simulink model "gm_fpga_block_pcie_slrt"  (R2020b)
settings: Solver=FixedStepDiscrete  StartTime=0.0  StopTime=5  FixedStep=5e-5  RelTol=1e-3
PostLoadFcn:
  | try
  | cell = struct2cell(dir(fullfile(speedgoatroot_hdlb, 'hdlsrc', 'quadrature', '*.vhd')));
  | addSourceFiles = strjoin(fullfile(cell(2,:),cell(1,:)), ';');
  | hdlset_param('quadrature_example_hdlc/DUT Quadrature', 'IPCoreAdditionalFiles', addSourceFiles);
  | end
undefined symbols (not defined in the file): FPGA, fpga_block, IO334
libraries: speedgoatlib_hdlCoder_IO3xx x19, eePwmGenerator x3, slrealtimeutilitieslib x1, pwm_cpulib x1, quadrature_cpulib x1
settings Model: ModifiedByFormat=Speedgoat GmbH  Creator=Speedgoat GmbH  LastModifiedBy=Speedgoat GmbH
settings SolverCC: ConcurrentTasks=on  PositivePriorityOrder=on
settings DataIOCC: ReturnWorkspaceOutputs=off
settings OptimizationCC: BlockReduction=off  ConditionallyExecuteInputs=off  DefaultParameterBehavior=Inlined  OptimizeBlockIOStorage=off
settings DebuggingCC: AlgebraicLoopMsg=error  InheritedTsInSrcMsg=none  SingleTaskRateTransMsg=error  TasksWithSamePriorityMsg=none  ParameterOverflowMsg=warning  ParameterPrecisionLossMsg=none  PregeneratedLibrarySubsystemCodeDiagnostic=none  ArithmeticOperatorsInVariantConditions=warning
settings HardwareCC: ProdBitPerLong=64  ProdLongLongMode=on  ProdHWDeviceType=Intel->x86-64 (Linux 64)  TargetBitPerPointer=64  TargetBitPerSizeT=64  TargetBitPerPtrDiffT=64  TargetLongLongMode=on  TargetIntDivRoundTo=Zero  TargetEndianess=LittleEndian  TargetWordSize=64  TargetHWDeviceType=Custom Processor->MATLAB Host Computer
settings SFSimCC: SimUseLocalCustomCode=off  CustomCodeUndefinedFunction=UseInterfaceOnly
settings RTWCC: Description=Simulink Real-Time  SystemTargetFile=slrealtime.tlc  TemplateMakefile=slrealtime_default_tmf  RTWUseLocalCustomCode=off  Toolchain=Simulink Real-Time Toolchain  BuildConfiguration=Faster Runs  CodeExecutionProfiling=on  TargetLang=C++

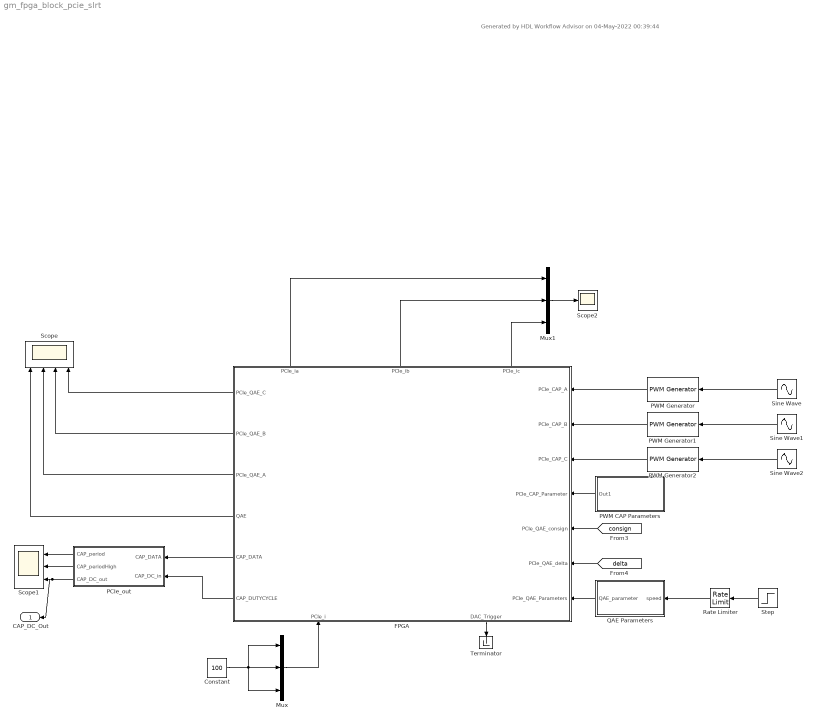
== system gm_fpga_block_pcie_slrt ==
  note: Generated by HDL Workflow Advisor on 04-May-2022 00:39:44
  Constant : Constant  Value=100  OutDataTypeStr=int16  SampleTime=5e-5
  FPGA : Subsystem  mask(Speedgoat IO334-325k Interface Block){module_id=1, slot=-1, ts=-1, FpgaFreq=100}
      mask prompts: module_id "FPGA Module Identifier:"; slot "PCI slot (-1: autosearch):"; ts "Sample time:"; FpgaFreq "FPGA Frequency [MHz]"
      mask help: Simulink Real-Time Interface Block for Speedgoat IO334-325k.
      mask init:
      | hdlslrt.backend.mfpgaparameters;
      settings: PortSchema="{\"entries\":[{\"content\":{\"sides\":[{\"content\":{\"connectorIds\":[\"In1\",\"In2\",\"In3\",\"In4\",\"In5\",\"In6\",\"In7\"]},\"type\":\"ConnectorPlacement.EquallySpacedRectSide\",\"uuid\":\"e6984190-0c70-4c87-a85a-93b5ecf8c70e\"},{\"content\":{\"connectorIds\":[\"Out1\",\"Out2\",\"Out3\",\"Out4\",\"Out5\",\"Out6\"],\"side\":\"RIGHT\"},\"type\":\"ConnectorPlacement.EquallySpacedRectSide\",\"uuid\":\"15751016-c591-4c93-a1ea-9b92ed7cff5f\"},{\"content\":{\"connectorIds\":[\"Out8\",\"Out9\",\"Out10\"],\"side\":\"TOP\"},\"type\":\"ConnectorPlacement.EquallySpacedRectSide\",\"uuid\":\"0ed2d626-9fdd-4a40-8e61-e2e65c1699d5\"},{\"content\":{\"connectorIds\":[\"Out7\",\"In8\"],\"side\":\"BOTTOM\"},\"type\":\"ConnectorPlacement.EquallySpacedRectSide\",\"uuid\":\"ca9e0c29-7634-4998-8fab-ad91c1afd2ab\"},{\"content\":{\"connectorIds\":[],\"side\":\"HIDDEN\"},\"type\":\"ConnectorPlacement.EquallySpacedRectSide\",\"uuid\":\"82c879c3-3b90-47c5-9b46-55d1ced3d9d8\"}]},\"type\":\"ConnectorPlacement.EquallySpacedConnector\",\"uuid\":\"f7068230-82ff-4dc7-8776-ae1c0daadd88\"}],\"packageUris\":[\"http://schema.mathworks.com/mf0/Connector/R2020b\"],\"version\":\"1.0\"}"
      mask Help: eval('speedgoatdoc_hdlc')
      mask Display:
      | SetupBlkPath = find_system(gcb, 'LookUnderMasks', 'all', 'FollowLinks', 'on', 'regexp', 'on', 'Name', 'IO3(\d|x){2}\s+Setup' );
      | SetupBlkPath = SetupBlkPath{1};
      | TS = get_param(SetupBlkPath,'timestamp_mcs');
      | disp(sprintf('Speedgoat IO334-325k\nFPGA I/O Module\n\nTimestamp\n%s\n\nReference Design\nVersion 2.1\n\nMatlab R2020b\n\nPCIe Link Width: X4\nRear Plugin: -21\nAurora Mode: None\nAurora Byteswap: true\n', TS))
  Mux : Mux  Inputs=3
  Mux1 : Mux  Inputs=3
  PCIe_out : Subsystem
  PWM CAP Parameters : Subsystem
  PWM Generator : eePwmGenerator/PWM Generator  CarrCount=Up  Tper=0.01  Ts=2e-4
  PWM Generator1 : eePwmGenerator/PWM Generator  CarrCount=Up  Tper=0.01  Ts=2e-4
  PWM Generator2 : eePwmGenerator/PWM Generator  CarrCount=Up  Tper=0.01  Ts=2e-4
  QAE Parameters : Subsystem
  Rate Limiter : RateLimiter  RisingSlewLimit=50  FallingSlewLimit=-50  SampleTimeMode=inherited
  Scope : Scope  NumInputPorts=4
  Scope1 : Scope  NumInputPorts=3
  Scope2 : Scope
  Sine Wave : Sin  Amplitude=0.5  Bias=0.5  Frequency=2*pi
  Sine Wave1 : Sin  Amplitude=0.5  Bias=0.5  Frequency=2*pi  Phase=2*pi/3
  Sine Wave2 : Sin  Amplitude=0.5  Bias=0.5  Frequency=2*pi  Phase=4*pi/3
  Step : Step  Time=0.1  After=100
  Terminator : Terminator
  CAP_DC_Out : Outport  VectorParamsAs1DForOutWhenUnconnected=off
  wires:
  Mux/1 -> FPGA/8(PCIe_i)
  FPGA/7(DAC_Trigger) -> Terminator/1
  FPGA/10(PCIe_ia) -> Mux1/1
  FPGA/9(PCIe_ib) -> Mux1/2
  FPGA/8(PCIe_ic) -> Mux1/3
  Mux1/1 -> Scope2/1
  Constant/1 -> Mux/1, Mux/2, Mux/3
  Sine Wave2/1 -> PWM Generator2/1
  Sine Wave1/1 -> PWM Generator1/1
  Sine Wave/1 -> PWM Generator/1
  Step/1 -> Rate Limiter/1
  Rate Limiter/1 -> QAE Parameters/1(speed)
  FPGA/6(CAP_DUTYCYCLE) -> PCIe_out/2(CAP_DC_in)
  FPGA/5(CAP_DATA) -> PCIe_out/1(CAP_DATA)
  FPGA/1(PCIe_QAE_C) -> Scope/4
  FPGA/2(PCIe_QAE_B) -> Scope/3
  FPGA/3(PCIe_QAE_A) -> Scope/2
  FPGA/4(QAE) -> Scope/1
  PWM CAP Parameters/1(Out1) -> FPGA/4(PCIe_CAP_Parameter)
  PWM Generator2/1 -> FPGA/3(PCIe_CAP_C)
  PWM Generator1/1 -> FPGA/2(PCIe_CAP_B)
  PWM Generator/1 -> FPGA/1(PCIe_CAP_A)
  [delta] -> FPGA/6(PCIe_QAE_delta)
  [consign] -> FPGA/5(PCIe_QAE_consign)
  QAE Parameters/1(QAE_parameter) -> FPGA/7(PCIe_QAE_Parameters)
  PCIe_out/3(CAP_DC_out) -> CAP_DC_Out/1, Scope1/3
  PCIe_out/2(CAP_periodHigh) -> Scope1/2
  PCIe_out/1(CAP_period) -> Scope1/1

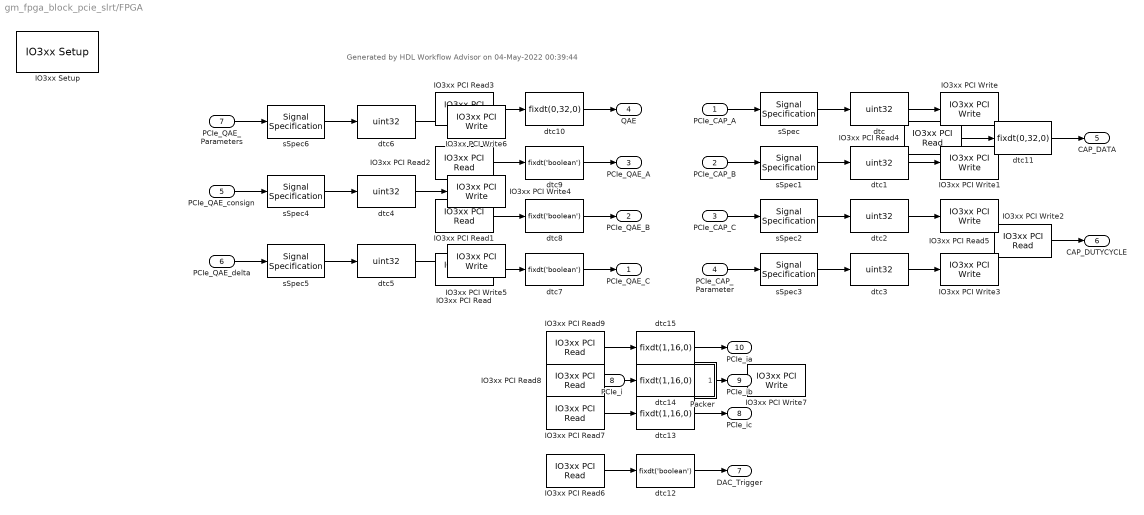
== system gm_fpga_block_pcie_slrt/FPGA ==
  note: Generated by HDL Workflow Advisor on 04-May-2022 00:39:44
  PCIe_CAP_A : Inport
  PCIe_CAP_B : Inport  Port=2
  PCIe_CAP_C : Inport  Port=3
  PCIe_CAP_Parameter : Inport  Port=4
  PCIe_QAE_consign : Inport  Port=5
  PCIe_QAE_delta : Inport  Port=6
  PCIe_QAE_Parameters : Inport  Port=7
  PCIe_i : Inport  Port=8
  IO3xx PCI Read : speedgoatlib_hdlCoder_IO3xx/IO3xx PCI Read  device_id=deviceIdx  module_id=module_id  board_type=IO3xx  port_name=PCIe_QAE_C  port_offset=hex2dec('164')  port_type=uint32  port_dim=1  strobe=0  sample_time=ts
  IO3xx PCI Read1 : speedgoatlib_hdlCoder_IO3xx/IO3xx PCI Read  device_id=deviceIdx  module_id=module_id  board_type=IO3xx  port_name=PCIe_QAE_B  port_offset=hex2dec('154')  port_type=uint32  port_dim=1  strobe=0  sample_time=ts
  IO3xx PCI Read2 : speedgoatlib_hdlCoder_IO3xx/IO3xx PCI Read  device_id=deviceIdx  module_id=module_id  board_type=IO3xx  port_name=PCIe_QAE_A  port_offset=hex2dec('13C')  port_type=uint32  port_dim=1  strobe=0  sample_time=ts
  IO3xx PCI Read3 : speedgoatlib_hdlCoder_IO3xx/IO3xx PCI Read  device_id=deviceIdx  module_id=module_id  board_type=IO3xx  port_name=QAE  port_offset=hex2dec('138')  port_type=uint32  port_dim=1  strobe=0  sample_time=ts
  IO3xx PCI Read4 : speedgoatlib_hdlCoder_IO3xx/IO3xx PCI Read  device_id=deviceIdx  module_id=module_id  board_type=IO3xx  port_name=CAP_DATA  port_offset=hex2dec('200')  port_type=uint32  port_dim=18  strobe=hex2dec('280')  sample_time=ts
  IO3xx PCI Read5 : speedgoatlib_hdlCoder_IO3xx/IO3xx PCI Read  device_id=deviceIdx  module_id=module_id  board_type=IO3xx  port_name=CAP_DUTYCYCLE  port_offset=hex2dec('170')  port_type=single  port_dim=3  strobe=hex2dec('180')  sample_time=ts
  IO3xx PCI Read6 : speedgoatlib_hdlCoder_IO3xx/IO3xx PCI Read  device_id=deviceIdx  module_id=module_id  board_type=IO3xx  port_name=DAC_Trigger  port_offset=hex2dec('184')  port_type=uint32  port_dim=1  strobe=0  sample_time=ts
  IO3xx PCI Read7 : speedgoatlib_hdlCoder_IO3xx/IO3xx PCI Read  device_id=deviceIdx  module_id=module_id  board_type=IO3xx  port_name=PCIe_ic  port_offset=hex2dec('168')  port_type=uint32  port_dim=1  strobe=0  sample_time=ts
  IO3xx PCI Read8 : speedgoatlib_hdlCoder_IO3xx/IO3xx PCI Read  device_id=deviceIdx  module_id=module_id  board_type=IO3xx  port_name=PCIe_ib  port_offset=hex2dec('16C')  port_type=uint32  port_dim=1  strobe=0  sample_time=ts
  IO3xx PCI Read9 : speedgoatlib_hdlCoder_IO3xx/IO3xx PCI Read  device_id=deviceIdx  module_id=module_id  board_type=IO3xx  port_name=PCIe_ia  port_offset=hex2dec('188')  port_type=uint32  port_dim=1  strobe=0  sample_time=ts
  IO3xx PCI Write : speedgoatlib_hdlCoder_IO3xx/IO3xx PCI Write  device_id=deviceIdx  module_id=module_id  board_type=IO3xx  port_name=PCIe_CAP_A  port_offset=hex2dec('12C')  port_type=uint32  port_dim=1  strobe=0  sample_time=ts
  IO3xx PCI Write1 : speedgoatlib_hdlCoder_IO3xx/IO3xx PCI Write  device_id=deviceIdx  module_id=module_id  board_type=IO3xx  port_name=PCIe_CAP_B  port_offset=hex2dec('130')  port_type=uint32  port_dim=1  strobe=0  sample_time=ts
  IO3xx PCI Write2 : speedgoatlib_hdlCoder_IO3xx/IO3xx PCI Write  device_id=deviceIdx  module_id=module_id  board_type=IO3xx  port_name=PCIe_CAP_C  port_offset=hex2dec('134')  port_type=uint32  port_dim=1  strobe=0  sample_time=ts
  IO3xx PCI Write3 : speedgoatlib_hdlCoder_IO3xx/IO3xx PCI Write  device_id=deviceIdx  module_id=module_id  board_type=IO3xx  port_name=PCIe_CAP_Parameter  port_offset=hex2dec('140')  port_type=uint32  port_dim=3  strobe=hex2dec('150')  sample_time=ts
  IO3xx PCI Write4 : speedgoatlib_hdlCoder_IO3xx/IO3xx PCI Write  device_id=deviceIdx  module_id=module_id  board_type=IO3xx  port_name=PCIe_QAE_consign  port_offset=hex2dec('124')  port_type=uint32  port_dim=1  strobe=0  sample_time=ts
  IO3xx PCI Write5 : speedgoatlib_hdlCoder_IO3xx/IO3xx PCI Write  device_id=deviceIdx  module_id=module_id  board_type=IO3xx  port_name=PCIe_QAE_delta  port_offset=hex2dec('128')  port_type=uint32  port_dim=1  strobe=0  sample_time=ts
  IO3xx PCI Write6 : speedgoatlib_hdlCoder_IO3xx/IO3xx PCI Write  device_id=deviceIdx  module_id=module_id  board_type=IO3xx  port_name=PCIe_QAE_Parameters  port_offset=hex2dec('100')  port_type=uint32  port_dim=7  strobe=hex2dec('120')  sample_time=ts
  IO3xx PCI Write7 : speedgoatlib_hdlCoder_IO3xx/IO3xx PCI Write  device_id=deviceIdx  module_id=module_id  board_type=IO3xx  port_name=PCIe_i  port_offset=hex2dec('158')  port_type=uint32  port_dim=2  strobe=hex2dec('160')  sample_time=ts
  IO3xx Setup : speedgoatlib_hdlCoder_IO3xx/IO3xx Setup  mdl_ss_name=fpga_block/FPGA  board_type=IO334-325k  fpga_sync_mode=on  reset_mode=on  device_id=deviceIdx  module_id=module_id  pci_slot=slot  fpga_mat_file=hdl_prj\hdlsrc\fpga_block\FPGA.mat  timestamp_mcs=mm/dd/yy HH:MM:SS  timestamp=2205031940  tsreg=hex2dec('8')  bsf_file=FPGA_2205031940.mcs  mcs=0
  Packer : Subsystem
  dtc{,1..6} (7 alike) : DataTypeConversion  OutDataTypeStr=uint32  ConvertRealWorld=Stored Integer (SI)  RndMeth=Zero
  dtc10 : DataTypeConversion  OutDataTypeStr=fixdt(0,32,0)  ConvertRealWorld=Stored Integer (SI)  RndMeth=Zero
  dtc11 : DataTypeConversion  OutDataTypeStr=fixdt(0,32,0)  ConvertRealWorld=Stored Integer (SI)  RndMeth=Zero
  dtc{7..9,12} (4 alike) : DataTypeConversion  OutDataTypeStr=fixdt('boolean')  ConvertRealWorld=Stored Integer (SI)  RndMeth=Zero
  dtc13 : DataTypeConversion  OutDataTypeStr=fixdt(1,16,0)  ConvertRealWorld=Stored Integer (SI)  RndMeth=Zero
  dtc14 : DataTypeConversion  OutDataTypeStr=fixdt(1,16,0)  ConvertRealWorld=Stored Integer (SI)  RndMeth=Zero
  dtc15 : DataTypeConversion  OutDataTypeStr=fixdt(1,16,0)  ConvertRealWorld=Stored Integer (SI)  RndMeth=Zero
  sSpec : SignalSpecification  OutDataTypeStr=fixdt('boolean')
  sSpec1 : SignalSpecification  OutDataTypeStr=fixdt('boolean')
  sSpec2 : SignalSpecification  OutDataTypeStr=fixdt('boolean')
  sSpec3 : SignalSpecification  OutDataTypeStr=fixdt(0,32,0)
  sSpec4 : SignalSpecification  OutDataTypeStr=fixdt(0,32,0)
  sSpec5 : SignalSpecification  OutDataTypeStr=fixdt(1,32,0)
  sSpec6 : SignalSpecification  OutDataTypeStr=fixdt(0,32,0)
  PCIe_QAE_C : Outport
  PCIe_QAE_B : Outport  Port=2
  PCIe_QAE_A : Outport  Port=3
  QAE : Outport  Port=4
  CAP_DATA : Outport  Port=5
  CAP_DUTYCYCLE : Outport  Port=6
  DAC_Trigger : Outport  Port=7
  PCIe_ic : Outport  Port=8
  PCIe_ib : Outport  Port=9
  PCIe_ia : Outport  Port=10
  wires:
  PCIe_CAP_A/1 -> sSpec/1
  sSpec/1 -> dtc/1
  dtc/1 -> IO3xx PCI Write/1
  PCIe_CAP_B/1 -> sSpec1/1
  sSpec1/1 -> dtc1/1
  dtc1/1 -> IO3xx PCI Write1/1
  PCIe_CAP_C/1 -> sSpec2/1
  sSpec2/1 -> dtc2/1
  dtc2/1 -> IO3xx PCI Write2/1
  PCIe_CAP_Parameter/1 -> sSpec3/1
  sSpec3/1 -> dtc3/1
  dtc3/1 -> IO3xx PCI Write3/1
  PCIe_QAE_consign/1 -> sSpec4/1
  sSpec4/1 -> dtc4/1
  dtc4/1 -> IO3xx PCI Write4/1
  PCIe_QAE_delta/1 -> sSpec5/1
  sSpec5/1 -> dtc5/1
  dtc5/1 -> IO3xx PCI Write5/1
  PCIe_QAE_Parameters/1 -> sSpec6/1
  sSpec6/1 -> dtc6/1
  dtc6/1 -> IO3xx PCI Write6/1
  PCIe_i/1 -> Packer/1(unpacked)
  Packer/1(packed) -> IO3xx PCI Write7/1
  dtc7/1 -> PCIe_QAE_C/1
  IO3xx PCI Read/1 -> dtc7/1
  dtc8/1 -> PCIe_QAE_B/1
  IO3xx PCI Read1/1 -> dtc8/1
  dtc9/1 -> PCIe_QAE_A/1
  IO3xx PCI Read2/1 -> dtc9/1
  dtc10/1 -> QAE/1
  IO3xx PCI Read3/1 -> dtc10/1
  dtc11/1 -> CAP_DATA/1
  IO3xx PCI Read4/1 -> dtc11/1
  IO3xx PCI Read5/1 -> CAP_DUTYCYCLE/1
  dtc12/1 -> DAC_Trigger/1
  IO3xx PCI Read6/1 -> dtc12/1
  dtc13/1 -> PCIe_ic/1
  IO3xx PCI Read7/1 -> dtc13/1
  dtc14/1 -> PCIe_ib/1
  IO3xx PCI Read8/1 -> dtc14/1
  dtc15/1 -> PCIe_ia/1
  IO3xx PCI Read9/1 -> dtc15/1

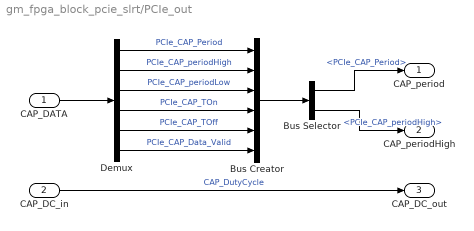
== system gm_fpga_block_pcie_slrt/PCIe_out ==
  CAP_DATA : Inport
  CAP_DC_in : Inport  Port=2
  Bus Creator : BusCreator  Inputs=6
  Bus Selector : BusSelector  OutputSignals=PCIe_CAP_Period,PCIe_CAP_periodHigh
  Demux : Demux  Outputs=6
  CAP_period : Outport
  CAP_periodHigh : Outport  Port=2
  CAP_DC_out : Outport  Port=3
  wires:
  CAP_DATA/1 -> Demux/1
  Demux/5 -> Bus Creator/5  "PCIe_CAP_TOff"
  Demux/1 -> Bus Creator/1  "PCIe_CAP_Period"
  Bus Creator/1 -> Bus Selector/1
  Demux/4 -> Bus Creator/4  "PCIe_CAP_TOn"
  Demux/2 -> Bus Creator/2  "PCIe_CAP_periodHigh"
  Demux/3 -> Bus Creator/3  "PCIe_CAP_periodLow"
  Demux/6 -> Bus Creator/6  "PCIe_CAP_Data_Valid"
  Bus Selector/1 -> CAP_period/1  "<PCIe_CAP_Period>"
  Bus Selector/2 -> CAP_periodHigh/1  "<PCIe_CAP_periodHigh>"
  CAP_DC_in/1 -> CAP_DC_out/1  "CAP_DutyCycle"

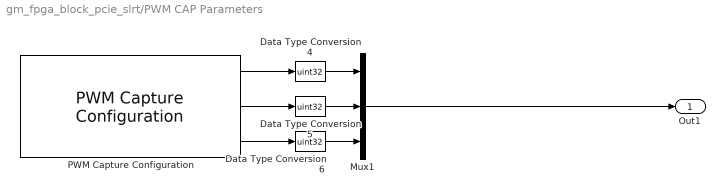
== system gm_fpga_block_pcie_slrt/PWM CAP Parameters ==
  Data Type Conversion4 : DataTypeConversion  OutDataTypeStr=uint32
  Data Type Conversion5 : DataTypeConversion  OutDataTypeStr=uint32
  Data Type Conversion6 : DataTypeConversion  OutDataTypeStr=uint32
  Mux1 : Mux  Inputs=3
  PWM Capture Configuration : pwm_cpulib/PWM Capture Configuration  FPGA_freq=100e6  n_channels=1  captureMode=High transitions triggered  captureTimeout=0  PWM_pattern_en=off
      settings: SourceProductName=Simulink Real-Time: Speedgoat HDL Blockset
  Out1 : Outport
  wires:
  Data Type Conversion5/1 -> Mux1/2
  PWM Capture Configuration/3 -> Data Type Conversion6/1
  Data Type Conversion4/1 -> Mux1/1
  PWM Capture Configuration/1 -> Data Type Conversion4/1
  Mux1/1 -> Out1/1
  Data Type Conversion6/1 -> Mux1/3
  PWM Capture Configuration/2 -> Data Type Conversion5/1

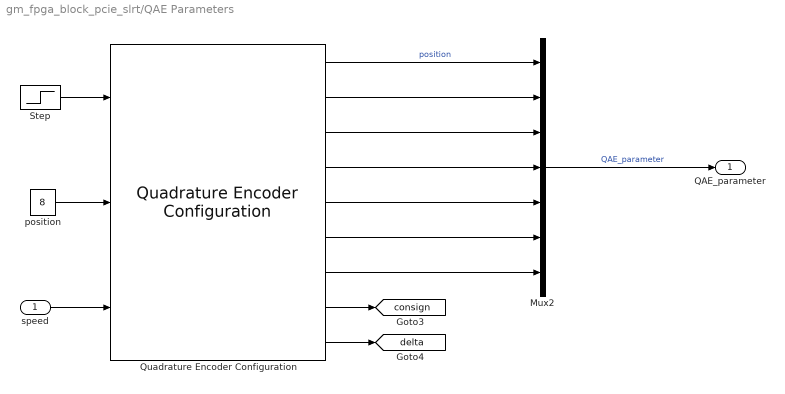
== system gm_fpga_block_pcie_slrt/QAE Parameters ==
  speed : Inport
  Mux2 : Mux  Inputs=7
  Quadrature Encoder Configuration : quadrature_cpulib/Quadrature Encoder Configuration  fpgaFreq=100e6  n_channels=1  numSeg=[16]  phaseAngle=90  initPos=[0]  freeWheel=on
      settings: SourceProductName=Simulink Real-Time: Speedgoat HDL Blockset
  Step : Step  Time=0.002
  position : Constant  Value=8  SampleTime=-1
  QAE_parameter : Outport
  tag scope: consign=global, delta=global
  wires:
  Mux2/1 -> QAE_parameter/1  "QAE_parameter"
  Quadrature Encoder Configuration/4 -> Mux2/4
  Quadrature Encoder Configuration/7 -> Mux2/7
  Step/1 -> Quadrature Encoder Configuration/1
  Quadrature Encoder Configuration/1 -> Mux2/1  "position"
  speed/1 -> Quadrature Encoder Configuration/3
  Quadrature Encoder Configuration/9 -> [delta]
  Quadrature Encoder Configuration/3 -> Mux2/3
  Quadrature Encoder Configuration/8 -> [consign]
  position/1 -> Quadrature Encoder Configuration/2
  Quadrature Encoder Configuration/6 -> Mux2/6
  Quadrature Encoder Configuration/5 -> Mux2/5
  Quadrature Encoder Configuration/2 -> Mux2/2

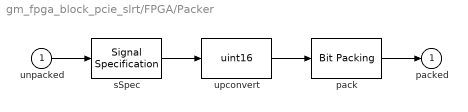
== system gm_fpga_block_pcie_slrt/FPGA/Packer ==
  unpacked : Inport
  pack : slrealtimeutilitieslib/Bit Packing  MaskBitPatterns={[0:15 16:31 32:47 ]}  MaskPackDataType=uint32  MaskPackDataSize=2
      settings: SourceProductBaseCode=XP
  sSpec : SignalSpecification  OutDataTypeStr=fixdt(1,16,0)
  upconvert : DataTypeConversion  OutDataTypeStr=uint16  ConvertRealWorld=Stored Integer (SI)  RndMeth=Zero
  packed : Outport
  wires:
  unpacked/1 -> sSpec/1
  sSpec/1 -> upconvert/1
  upconvert/1 -> pack/1
  pack/1 -> packed/1
